simulink model "simcourbe"  (R2018a)
settings: Solver=VariableStepAuto  StartTime=0.0  StopTime=10.0  RelTol=1e-3
undefined symbols (not defined in the file): sigbuilder_block
settings Model: Creator=Raval  LastModifiedBy=Raval

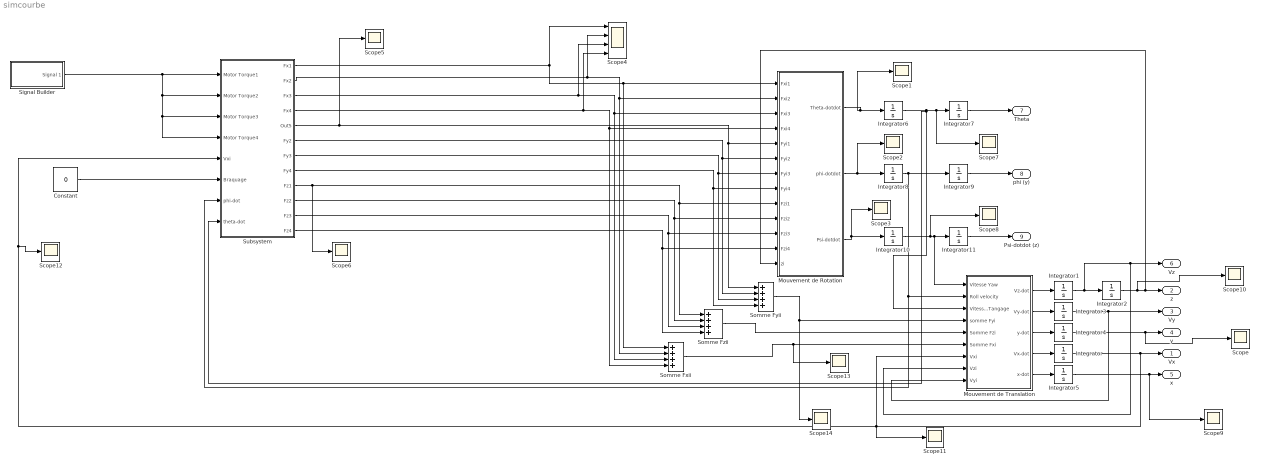
== system simcourbe ==
  Constant : Constant  Value=0  VectorParams1D=off  SampleTime=-1
  Integrator{,1..11} (12 alike) : Integrator
  Mouvement de Rotation : Subsystem
  Mouvement de Translation : Subsystem
  Scope{,1..3,5..14} (14 alike) : Scope
  Scope4 : Scope  NumInputPorts=4
  Signal Builder : Subsystem  Tag=STV Subsys  LoadFcn=sigbuilder_block('load');  StartFcn=sigbuilder_block('start');  StopFcn=sigbuilder_block('stop');  ClipboardFcn=sigbuilder_block('clipboard');  mask(Sigbuilder block){tuvar=[0:10]}
      mask help: Simulink:masks:SigbuilderBlock_MD
      mask init:
      | if ~strcmp(get_param(bdroot(gcbh),'SimulationStatus'),'stopped') tuvar = sigbuilder_block('maskInit'); end
      settings: CopyFcn=sigbuilder_block('copy');  DeleteFcn=sigbuilder_block('delete');  ModelCloseFcn=sigbuilder_block('modelClose');  PreSaveFcn=sigbuilder_block('preSave');  PauseFcn=sigbuilder_block('pause');  ContinueFcn=sigbuilder_block('continue');  NameChangeFcn=sigbuilder_block('namechange');  OpenFcn=sigbuilder_block('open',[366.6 79.8 550.8 400.2 ]);  CloseFcn=sigbuilder_block('close');
      mask Display: plot(0, 0, 100, 100,[2, 2, 32, 32, 2], [68, 8, 8, 68, 68],[32, 2], [38, 38], [32, 19, 2],[53, 60, 44], [32, 17, 17, 2],[16, 16, 31, 31]);txt = getActiveGroup(gcbh);text(2, 100, txt,'verticalAlignment', 'top');
  Somme Fxii : Sum  Inputs=++++
  Somme Fyii : Sum  Inputs=++++
  Somme Fzii : Sum  Inputs=++++
  Subsystem : Subsystem
  Vx : Outport
  z : Outport  Port=2
  Vy : Outport  Port=3
  y : Outport  Port=4
  x : Outport  Port=5
  Vz : Outport  Port=6
  Theta : Outport  Port=7
  phi (y) : Outport  Port=8
  Psi-dotdot (z) : Outport  Port=9
  wires:
  Integrator9/1 -> phi (y)/1
  Subsystem/4(Fx4) -> Scope4/4, Somme Fxii/4, Mouvement de Rotation/4(Fxi4)
  Signal Builder/1(Signal 1) -> Subsystem/1(Motor Torque1), Subsystem/2(Motor Torque2), Subsystem/3(Motor Torque3), Subsystem/4(Motor Torque4)
  Integrator4/1 -> Scope/1, y/1
  Integrator5/1 -> Scope9/1, x/1
  Subsystem/11(Fz3) -> Somme Fzii/3, Mouvement de Rotation/11(Fzi3)
  Subsystem/1(Fx1) -> Mouvement de Rotation/1(Fxi1), Somme Fxii/1, Scope4/1
  Integrator1/1 -> Mouvement de Translation/8(Vzi), Vz/1, Integrator2/1
  Subsystem/3(Fx3) -> Scope4/3, Mouvement de Rotation/3(Fxi3), Somme Fxii/3
  Mouvement de Translation/2(Vy-dot) -> Integrator3/1
  Integrator2/1 -> Scope10/1, Mouvement de Rotation/13(zi), z/1
  Subsystem/5(Out5) -> Scope5/1, Somme Fyii/1, Mouvement de Rotation/5(Fyi1)
  Mouvement de Translation/1(Vz-dot) -> Integrator1/1
  Subsystem/2(Fx2) -> Scope4/2, Somme Fxii/2, Mouvement de Rotation/2(Fxi2)
  Mouvement de Rotation/3(Psi-dotdot) -> Scope3/1, Integrator10/1
  Mouvement de Rotation/1(Theta-dotdot) -> Scope1/1, Integrator6/1
  Subsystem/9(Fz1) -> Scope6/1, Mouvement de Rotation/9(Fzi1), Somme Fzii/1
  Subsystem/6(Fy2) -> Somme Fyii/2, Mouvement de Rotation/6(Fyi2)
  Mouvement de Translation/5(x-dot) -> Integrator5/1
  Somme Fzii/1 -> Mouvement de Translation/5(Somme Fzi)
  Subsystem/10(Fz2) -> Somme Fzii/2, Mouvement de Rotation/10(Fzi2)
  Subsystem/7(Fy3) -> Mouvement de Rotation/7(Fyi3), Somme Fyii/3
  Mouvement de Translation/4(Vx-dot) -> Integrator/1
  Integrator10/1 -> Scope8/1, Mouvement de Translation/1(Vitesse Yaw), Integrator11/1
  Integrator11/1 -> Psi-dotdot (z)/1
  Subsystem/12(Fz4) -> Somme Fzii/4, Mouvement de Rotation/12(Fzi4)
  Integrator8/1 -> Subsystem/7(phi-dot), Mouvement de Translation/2(Roll velocity), Integrator9/1
  Integrator3/1 -> Vy/1, Mouvement de Translation/9(Vyi)
  Mouvement de Translation/3(y-dot) -> Integrator4/1
  Subsystem/8(Fy4) -> Somme Fyii/4, Mouvement de Rotation/8(Fyi4)
  Somme Fyii/1 -> Scope14/1, Mouvement de Translation/4(somme Fyi)
  Integrator7/1 -> Theta/1
  Integrator/1 -> Scope12/1, Subsystem/5(Vxi), Scope11/1, Mouvement de Translation/7(Vxi), Vx/1
  Integrator6/1 -> Subsystem/8(theta-dot), Mouvement de Translation/3(Vitesse Tangage), Scope7/1, Integrator7/1
  Constant/1 -> Subsystem/6(Braquage)
  Mouvement de Rotation/2(phi-dotdot) -> Scope2/1, Integrator8/1
  Somme Fxii/1 -> Scope13/1, Mouvement de Translation/6(Somme Fxi)

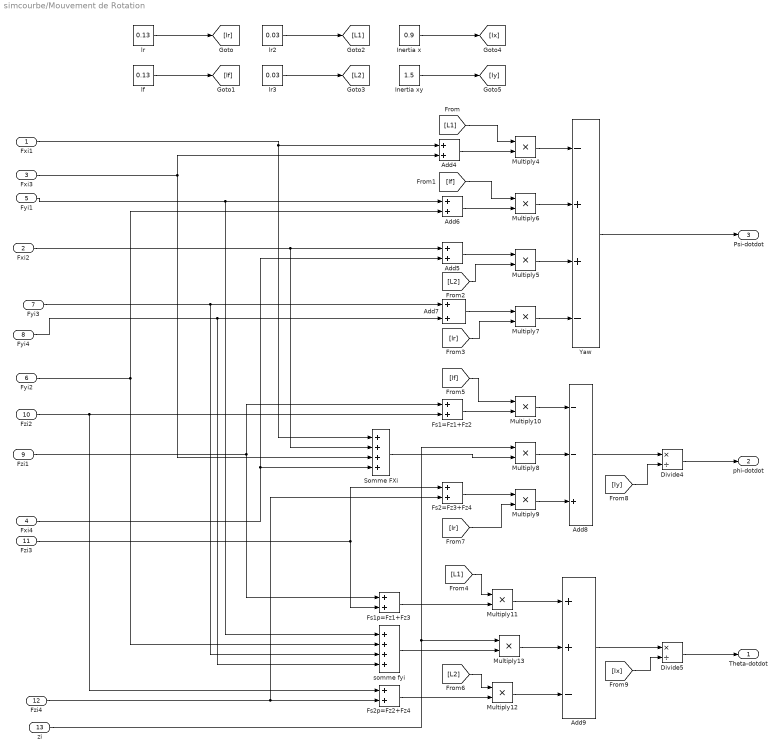
== system simcourbe/Mouvement de Rotation ==
  Fxi1 : Inport
  Fxi2 : Inport  Port=2
  Fxi3 : Inport  Port=3
  Fxi4 : Inport  Port=4
  Fyi1 : Inport  Port=5
  Fyi2 : Inport  Port=6
  Fyi3 : Inport  Port=7
  Fyi4 : Inport  Port=8
  Fzi1 : Inport  Port=9
  Fzi2 : Inport  Port=10
  Fzi3 : Inport  Port=11
  Fzi4 : Inport  Port=12
  zi : Inport  Port=13
  Add{4..7} (4 alike) : Sum
  Add8 : Sum  Inputs=--+
  Add9 : Sum  Inputs=++-
  Divide4 : Product  Inputs=*/
  Divide5 : Product  Inputs=*/
  Fs1=Fz1+Fz2 : Sum
  Fs1p=Fz1+Fz3 : Sum
  Fs2=Fz3+Fz4 : Sum
  Fs2p=Fz2+Fz4 : Sum
  Inertia x : Constant  Value=0.9
  Inertia xy : Constant  Value=1.5
  Multiply{4..13} (10 alike) : Product
  Somme FXi : Sum  Inputs=++++
  Yaw : Sum  Inputs=-++-
  lf : Constant  Value=0.13
  lr : Constant  Value=0.13
  lr2 : Constant  Value=0.03
  lr3 : Constant  Value=0.03
  somme fyi : Sum  Inputs=++++
  Theta-dotdot : Outport
  phi-dotdot : Outport  Port=2
  Psi-dotdot : Outport  Port=3
  wires:
  Add9/1 -> Divide5/1
  Fxi3/1 -> Add4/2, Somme FXi/3
  Yaw/1 -> Psi-dotdot/1
  Multiply9/1 -> Add8/3
  Fxi1/1 -> Somme FXi/1, Add4/1
  zi/1 -> Multiply8/1, Multiply13/1
  Fs2=Fz3+Fz4/1 -> Multiply9/1
  Fyi1/1 -> somme fyi/1, Add6/1
  Fs1p=Fz1+Fz3/1 -> Multiply11/2
  Divide4/1 -> phi-dotdot/1
  Multiply10/1 -> Add8/1
  Add8/1 -> Divide4/1
  Fyi2/1 -> Add6/2, somme fyi/2
  Fxi4/1 -> Add5/2, Somme FXi/4
  Fzi1/1 -> Fs1p=Fz1+Fz3/1, Fs1=Fz1+Fz2/1
  [lr] -> Multiply7/2
  Multiply8/1 -> Add8/2
  Fzi3/1 -> Fs1p=Fz1+Fz3/2, Fs2=Fz3+Fz4/1
  [L2] -> Multiply5/2
  Multiply12/1 -> Add9/3
  Fyi3/1 -> somme fyi/3, Add7/1
  Fxi2/1 -> Somme FXi/2, Add5/1
  [Ix] -> Divide5/2
  somme fyi/1 -> Multiply13/2
  Add5/1 -> Multiply5/1
  Fzi2/1 -> Fs2p=Fz2+Fz4/1, Fs1=Fz1+Fz2/2
  Divide5/1 -> Theta-dotdot/1
  Fyi4/1 -> somme fyi/4, Add7/2
  [lr] -> Multiply9/2
  Fzi4/1 -> Fs2=Fz3+Fz4/2, Fs2p=Fz2+Fz4/2
  [Iy] -> Divide4/2
  Fs1=Fz1+Fz2/1 -> Multiply10/2
  [lf] -> Multiply10/1
  Multiply13/1 -> Add9/2
  Multiply6/1 -> Yaw/2
  Somme FXi/1 -> Multiply8/2
  [L1] -> Multiply11/1
  Fs2p=Fz2+Fz4/1 -> Multiply12/2
  Multiply4/1 -> Yaw/1
  Multiply7/1 -> Yaw/4
  [L2] -> Multiply12/1
  Multiply11/1 -> Add9/1
  Add7/1 -> Multiply7/1
  Multiply5/1 -> Yaw/3
  lr/1 -> [lr]
  lf/1 -> [lf]
  lr2/1 -> [L1]
  lr3/1 -> [L2]
  Inertia x/1 -> [Ix]
  Inertia xy/1 -> [Iy]
  Add4/1 -> Multiply4/2
  [L1] -> Multiply4/1
  Add6/1 -> Multiply6/2
  [lf] -> Multiply6/1

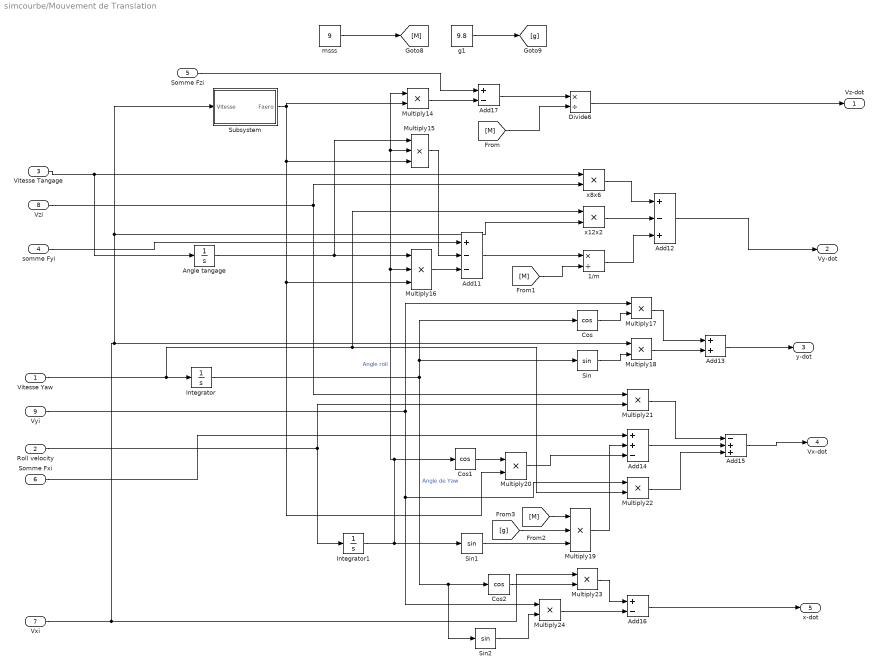
== system simcourbe/Mouvement de Translation ==
  Vitesse Yaw : Inport
  Roll velocity : Inport  Port=2
  Vitesse Tangage : Inport  Port=3
  somme Fyi : Inport  Port=4
  Somme Fzi : Inport  Port=5
  Somme Fxi : Inport  Port=6
  Vxi : Inport  Port=7
  Vzi : Inport  Port=8
  Vyi : Inport  Port=9
  1/m : Product  Inputs=*/
  Add11 : Sum  Inputs=+--
  Add12 : Sum  Inputs=+-+
  Add13 : Sum
  Add14 : Sum  Inputs=++-
  Add15 : Sum  Inputs=-++
  Add16 : Sum  Inputs=+-
  Add17 : Sum  Inputs=+-
  Angle tangage : Integrator
  Cos : Trigonometry  Operator=cos
  Cos1 : Trigonometry  Operator=cos
  Cos2 : Trigonometry  Operator=cos
  Divide6 : Product  Inputs=*/
  Integrator : Integrator
  Integrator1 : Integrator
  Multiply{14,17..18,20..24} (8 alike) : Product
  Multiply15 : Product  Inputs=3
  Multiply16 : Product  Inputs=3
  Multiply19 : Product  Inputs=3
  Sin : Trigonometry
  Sin1 : Trigonometry
  Sin2 : Trigonometry
  Subsystem : Subsystem
  g1 : Constant  Value=9.8
  msss : Constant  Value=9
  x12x2 : Product
  x8x6 : Product
  Vz-dot : Outport
  Vy-dot : Outport  Port=2
  y-dot : Outport  Port=3
  Vx-dot : Outport  Port=4
  x-dot : Outport  Port=5
  wires:
  Vzi/1 -> x8x6/2, Multiply21/1
  Vitesse Yaw/1 -> x12x2/1, Multiply22/2, Integrator/1
  Multiply23/1 -> Add16/1
  Add12/1 -> Vy-dot/1
  Roll velocity/1 -> Multiply21/2, Integrator1/1
  Vyi/1 -> Multiply24/1, Multiply22/1, Multiply17/1
  Add17/1 -> Divide6/1
  somme Fyi/1 -> Add11/1
  Multiply14/1 -> Add17/2
  Subsystem/1(Faero) -> Multiply14/2, Multiply20/2, Multiply16/3, Multiply15/3
  Add15/1 -> Vx-dot/1
  Somme Fzi/1 -> Add17/1
  Integrator/1 -> Sin2/1, Cos2/1, Cos/1, Sin/1  "Angle de Yaw"
  Multiply18/1 -> Add13/2
  Vxi/1 -> Multiply23/1, Subsystem/1(Vitesse), x12x2/2, Multiply18/1
  Integrator1/1 -> Multiply14/1, Multiply15/2, Multiply16/2, Cos1/1, Sin1/1  "Angle roll"
  Add11/1 -> 1/m/1
  Multiply19/1 -> Add14/2
  Multiply24/1 -> Add16/2
  Add14/1 -> Add15/2
  Vitesse Tangage/1 -> Angle tangage/1, x8x6/1
  Angle tangage/1 -> Multiply15/1, Multiply16/1
  Sin2/1 -> Multiply24/2
  Multiply22/1 -> Add15/3
  Add16/1 -> x-dot/1
  Somme Fxi/1 -> Add14/1
  [M] -> Divide6/2
  Multiply16/1 -> Add11/3
  Add13/1 -> y-dot/1
  1/m/1 -> Add12/3
  Divide6/1 -> Vz-dot/1
  Sin/1 -> Multiply18/2
  x12x2/1 -> Add12/2
  Cos/1 -> Multiply17/2
  Multiply17/1 -> Add13/1
  Cos1/1 -> Multiply20/1
  Multiply20/1 -> Add14/3
  Multiply15/1 -> Add11/2
  x8x6/1 -> Add12/1
  Cos2/1 -> Multiply23/2
  Multiply21/1 -> Add15/1
  Sin1/1 -> Multiply19/3
  [g] -> Multiply19/2
  msss/1 -> [M]
  [M] -> 1/m/2
  [M] -> Multiply19/1
  g1/1 -> [g]

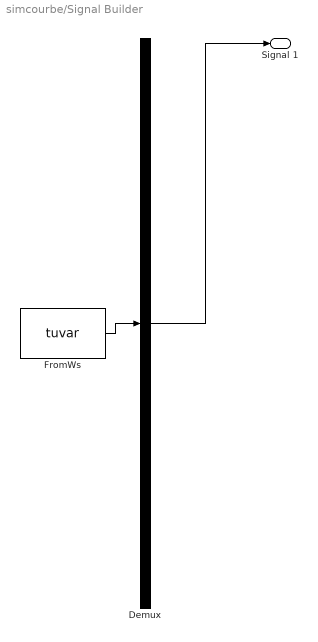
== system simcourbe/Signal Builder ==
  Demux : Demux  Tag=STV Demux  Outputs=1
  FromWs : FromWorkspace  Tag=STV FromWs  VariableName=tuvar  SampleTime=0
      SigBuilderData=|
      | common.afterFinalStr = 'Extrapolate'
      | common.sampleTime = 0
      | dataSet.timeRange = [0 10]
      | dataSet.name = 'Group 1'
      | sbobj.Groups.Name = 'Group 1'
      | sbobj.Groups.Signals.Name = 'Signal 1'
      | sbobj.Groups.Signals.XData = [0 4 4 6 6 10]
      | sbobj.Groups.Signals.YData = [0 0.995 1 1 0.995 0.995]
  Signal 1 : Outport  Tag=STV Outport
  wires:
  Demux/1 -> Signal 1/1
  FromWs/1 -> Demux/1

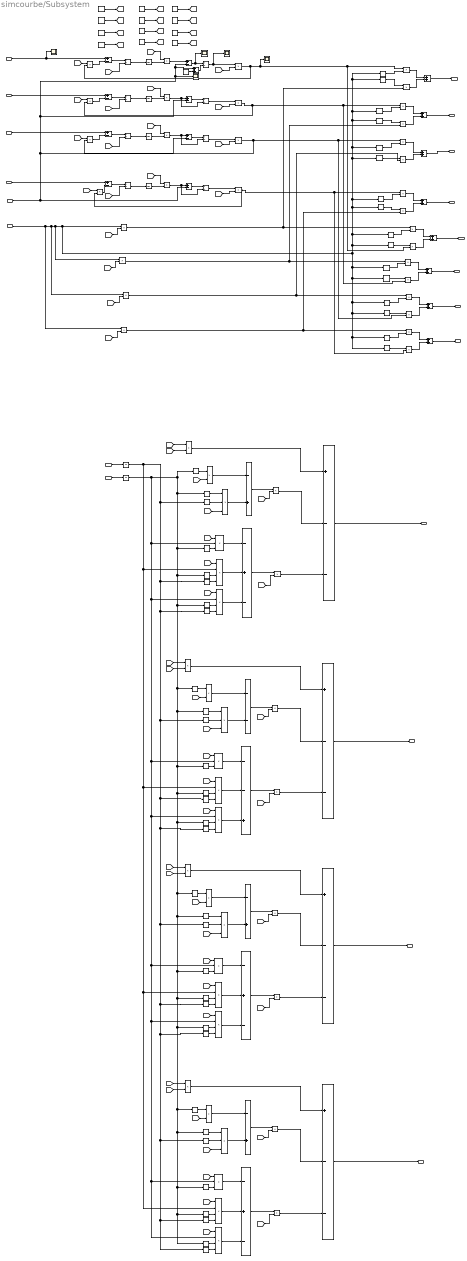
== system simcourbe/Subsystem ==
  Motor Torque1 : Inport
  Motor Torque2 : Inport  Port=2
  Motor Torque3 : Inport  Port=3
  Motor Torque4 : Inport  Port=4
  Vxi : Inport  Port=5
  Braquage : Inport  Port=6
  phi-dot : Inport  Port=7
  theta-dot : Inport  Port=8
  Add{,5..11,24} (9 alike) : Sum
  Add{1..4} (4 alike) : Sum  Inputs=+-
  Add12 : Sum  Inputs=-+
  Add13 : Sum  Inputs=-+-
  Add{14,17,20,23} (4 alike) : Sum  Inputs=+--
  Add15 : Sum  Inputs=--
  Add16 : Sum  Inputs=--+
  Add18 : Sum  Inputs=-+
  Add19 : Sum  Inputs=-+-
  Add21 : Sum  Inputs=-+
  Add22 : Sum  Inputs=-+-
  Coefficient Fx : Constant  Value=0.1
  Constant : Constant  Value=0.1
  Constant1 : Constant  Value=0.5
  Constant2 : Constant  Value=0.000001
  Cos{,1..11,14..15,18..21,24..27,30..31} (24 alike) : Trigonometry  Operator=cos
  Cos{12..13,16..17,22..23,28..29} (8 alike) : Trigonometry
  Divide{2..9} (8 alike) : Product  Inputs=*/
  Inertia Roue : Constant  Value=0.2
  Integrator : Integrator
  Integrator12 : Integrator
  Integrator14 : Integrator  InitialCondition=0.001
  Integrator15 : Integrator  InitialCondition=0.001
  Integrator16 : Integrator  InitialCondition=0.001
  Integrator17 : Integrator
  Kvi : Constant
  L1 : Constant  Value=0.03
  L2 : Constant  Value=0.03
  Multiply{,1..24,26,30..32,34,38..40,42,46..48,50,54..59} (44 alike) : Product
  Multiply{25,27,33,35,41,43,49,51} (8 alike) : Product  Inputs=3
  Multiply{28..29,36..37,44..45,52..53} (8 alike) : Product  Inputs=4
  Rayon : Constant  Value=0.031
  Rw-vx{1..4} (4 alike) : Sum  Inputs=+-
  Rw{1..4} (4 alike) : Product
  Scope{,1..2,4..5} (5 alike) : Scope
  Sin{,1..15} (16 alike) : Trigonometry
  g : Constant  Value=9.8
  ksi : Constant
  lf : Constant  Value=0.13
  lr : Constant  Value=0.13
  Fx1 : Outport
  Fx2 : Outport  Port=2
  Fx3 : Outport  Port=3
  Fx4 : Outport  Port=4
  Out5 : Outport  Port=5
  Fy2 : Outport  Port=6
  Fy3 : Outport  Port=7
  Fy4 : Outport  Port=8
  Fz1 : Outport  Port=9
  Fz2 : Outport  Port=10
  Fz3 : Outport  Port=11
  Fz4 : Outport  Port=12
  wires:
  Integrator17/1 -> Multiply53/2, Multiply51/2, Multiply45/2, Multiply43/2, Multiply37/2, Multiply35/2, Multiply29/2, Multiply27/2, Cos9/1, Cos28/1, Cos26/1, Cos31/1, Cos30/1, Sin14/1, Cos22/1, Cos20/1, Cos25/1, Cos24/1, Sin12/1, Cos16/1, Cos14/1, Cos19/1, Cos18/1, Sin10/1, Cos12/1, Cos10/1, Cos8/1, Sin8/1
  Multiply12/1 -> Add6/1
  Integrator12/1 -> Multiply52/2, Multiply44/2, Multiply36/2, Multiply28/2, Cos11/1, Cos13/1, Cos15/1, Cos17/1, Cos21/1, Cos23/1, Cos29/1, Cos27/1, Sin15/1, Sin13/1, Sin11/1, Sin9/1
  Add8/1 -> Out5/1
  Sin9/1 -> Multiply25/2
  Add4/1 -> Divide8/1
  Multiply35/1 -> Add16/1
  Divide4/1 -> Integrator14/1
  [Cy] -> Multiply6/2
  Vxi/1 -> Rw-vx4/2, Rw-vx2/2, Add24/1, Rw-vx1/2, Scope2/1, Rw-vx3/2
  Rw-vx2/1 -> Divide5/1
  Braquage/1 -> Multiply7/1, Multiply6/1, Multiply5/1, Sin3/1, Cos/1, Sin/1, Cos1/1, Sin1/1, Cos2/1, Sin2/1, Cos3/1, Cos4/1, Sin4/1, Sin7/1, Cos7/1, Sin6/1, Cos6/1, Sin5/1, Cos5/1, Multiply/1
  Multiply8/1 -> Add/1
  Multiply55/1 -> Add23/2
  Add6/1 -> Fx3/1
  Cos24/1 -> Multiply41/1
  [Cx] -> Multiply3/2
  Add13/1 -> Multiply30/1
  [L2] -> Multiply37/1
  Cos17/1 -> Multiply37/4
  Constant1/1 -> [M]
  Sin/1 -> Multiply9/1
  Sin14/1 -> Multiply50/1
  Rw2/1 -> Divide5/2, Rw-vx2/1
  Multiply18/1 -> Add9/1
  Multiply22/1 -> Add11/1
  Divide8/1 -> Integrator16/1
  Sin7/1 -> Multiply23/1
  Integrator15/1 -> Rw3/2
  Cos30/1 -> Multiply49/1
  Add/1 -> Fx1/1
  Sin1/1 -> Multiply11/1
  Cos2/1 -> Multiply12/2
  Integrator16/1 -> Rw4/2
  Cos6/1 -> Multiply20/2
  L2/1 -> [L2]
  [L1] -> Multiply45/1
  Multiply45/1 -> Add19/3
  Integrator14/1 -> Rw2/2
  Cos3/1 -> Multiply14/2
  [R] -> Rw3/1
  Multiply10/1 -> Add5/1
  Divide9/1 -> Multiply4/1
  Sin10/1 -> Multiply34/1
  Add20/1 -> Fz3/1
  Multiply51/1 -> Add22/1
  [L1] -> Multiply28/1
  Multiply1/1 -> Multiply56/2, Scope1/1, Multiply17/2, Multiply8/1  "Fxpi"
  [Cy] -> Multiply/2
  Add17/1 -> Fz2/1
  Add23/1 -> Fz4/1
  Multiply27/1 -> Add13/1
  Rw4/1 -> Divide9/2, Rw-vx4/1
  [M] -> Multiply48/2
  Multiply7/1 -> Multiply22/1, Multiply15/2  "Fypi"
  Motor Torque2/1 -> Add2/1
  Multiply24/1 -> Add14/1
  theta-dot/1 -> Integrator12/1
  Kvi/1 -> [kvi]
  phi-dot/1 -> Integrator17/1
  Rayon/1 -> [R]
  [Ir] -> Divide8/2
  [Cy] -> Multiply7/2
  Constant/1 -> [Cy]
  Integrator/1 -> Rw1/2
  Cos11/1 -> Multiply28/4
  Add5/1 -> Fx2/1
  Add14/1 -> Fz1/1
  Cos7/1 -> Multiply22/2
  Rw3/1 -> Divide7/2, Rw-vx3/1
  Divide7/1 -> Multiply3/1
  [R] -> Rw1/1
  ksi/1 -> [ksi]
  Rw-vx1/1 -> Scope5/1, Divide3/1
  Sin5/1 -> Multiply19/1
  [Ir] -> Divide2/2
  [ksi] -> Multiply55/2
  Divide3/1 -> Scope4/1, Multiply1/1
  [R] -> Rw2/1
  Multiply/1 -> Multiply16/1, Multiply9/2  "Fypi"
  Inertia Roue/1 -> [Ir]
  Multiply17/1 -> Add8/2
  Cos18/1 -> Multiply33/1
  Rw-vx3/1 -> Divide7/1
  Multiply13/1 -> Add6/2
  Multiply54/1 -> Add23/3
  [kvi] -> Multiply46/2
  Multiply44/1 -> Add19/2
  Motor Torque3/1 -> Add3/1
  Rw-vx4/1 -> Divide9/1
  Multiply30/1 -> Add14/3
  Add22/1 -> Multiply54/1
  Cos13/1 -> Multiply29/4
  Add7/1 -> Fx4/1
  [ksi] -> Multiply31/2
  Multiply21/1 -> Add10/2
  Multiply47/1 -> Add20/2
  Add1/1 -> Divide2/1
  [lf] -> Multiply27/1
  Cos28/1 -> Multiply53/3
  Cos29/1 -> Multiply53/4
  Multiply6/1 -> Multiply20/1, Multiply13/2  "Fypi"
  Multiply11/1 -> Add5/2
  Cos20/1 -> Multiply44/3
  [Cx] -> Multiply2/2
  [L2] -> Multiply52/1
  L1/1 -> [L1]
  Cos23/1 -> Multiply45/4
  Cos26/1 -> Multiply52/3
  Multiply28/1 -> Add13/2
  Multiply16/1 -> Add8/1
  Cos9/1 -> Multiply27/3
  Cos5/1 -> Multiply18/2
  Add15/1 -> Multiply39/1
  Cos10/1 -> Multiply28/3
  Cos19/1 -> Multiply35/3
  Cos16/1 -> Multiply37/3
  [lf] -> Multiply35/1
  lf/1 -> [lf]
  Multiply31/1 -> Add14/2
  [kvi] -> Multiply38/2
  [L1] -> Multiply25/3
  Sin3/1 -> Multiply15/1
  Multiply32/1 -> Add17/1
  [Cx] -> Multiply4/2
  Multiply38/1 -> Add17/3
  Cos31/1 -> Multiply51/3
  Multiply37/1 -> Add16/3
  Coefficient Fx/1 -> [Cx]
  Sin4/1 -> Multiply17/1
  Multiply19/1 -> Add9/2
  Sin11/1 -> Multiply33/2
  [L2] -> Multiply49/3
  Add10/1 -> Fy3/1
  [R] -> Rw4/1
  Multiply5/1 -> Multiply18/1, Multiply11/2  "Fypi"
  [ksi] -> Multiply39/2
  Multiply29/1 -> Add13/3
  Multiply23/1 -> Add11/2
  [M] -> Multiply32/2
  [kvi] -> Multiply30/2
  Multiply36/1 -> Add16/2
  Multiply39/1 -> Add17/2
  [M] -> Multiply40/2
  [Ir] -> Divide6/2
  Motor Torque4/1 -> Add4/1
  [g] -> Multiply40/1
  [L1] -> Multiply41/3
  [lr] -> Multiply42/2
  Sin6/1 -> Multiply21/1
  Cos15/1 -> Multiply36/4
  Divide2/1 -> Integrator/1
  Add12/1 -> Multiply31/1
  [L1] -> Multiply29/1
  Multiply34/1 -> Add15/1
  Multiply48/1 -> Add23/1
  Sin12/1 -> Multiply42/1
  Multiply46/1 -> Add20/3
  [Ir] -> Divide4/2
  Sin13/1 -> Multiply41/2
  Multiply41/1 -> Add18/2
  [Cy] -> Multiply5/2
  Multiply42/1 -> Add18/1
  Cos25/1 -> Multiply43/3
  Add2/1 -> Divide4/1
  Cos4/1 -> Multiply16/2
  [L2] -> Multiply33/3
  [lf] -> Multiply43/1
  Multiply40/1 -> Add20/1
  Cos21/1 -> Multiply44/4
  Cos12/1 -> Multiply29/3
  [ksi] -> Multiply47/2
  [L2] -> Multiply53/1
  Cos14/1 -> Multiply36/3
  [g] -> Multiply48/1
  Multiply20/1 -> Add10/1
  Divide5/1 -> Multiply2/1
  Cos22/1 -> Multiply45/3
  Add3/1 -> Divide6/1
  [L2] -> Multiply36/1
  [L1] -> Multiply44/1
  Multiply53/1 -> Add22/3
  Add18/1 -> Multiply47/1
  Multiply50/1 -> Add21/1
  Multiply49/1 -> Add21/2
  [lr] -> Multiply50/2
  [kvi] -> Multiply54/2
  Sin15/1 -> Multiply49/2
  lr/1 -> [lr]
  [g] -> Multiply32/1
  Add21/1 -> Multiply55/1
  Multiply33/1 -> Add15/2
  Multiply15/1 -> Add7/2
  Add16/1 -> Multiply38/1
  Add19/1 -> Multiply46/1
  [lf] -> Multiply51/1
  Multiply43/1 -> Add19/1
  [lf] -> Multiply34/2
  [Cx] -> Multiply1/2
  Divide6/1 -> Integrator15/1
  Cos8/1 -> Multiply25/1
  Multiply52/1 -> Add22/2
  Multiply9/1 -> Add/2
  Cos27/1 -> Multiply52/4
  Multiply25/1 -> Add12/2
  Multiply14/1 -> Add7/1
  Cos1/1 -> Multiply10/2
  Cos/1 -> Multiply8/2
  Add11/1 -> Fy4/1
  Sin2/1 -> Multiply13/1
  Add9/1 -> Fy2/1
  [M] -> Multiply24/2
  Multiply26/1 -> Add12/1
  [g] -> Multiply24/1
  g/1 -> [g]
  Sin8/1 -> Multiply26/1
  [lf] -> Multiply26/2
  Motor Torque1/1 -> Scope/1, Add1/1
  Multiply56/1 -> Add1/2
  [R] -> Multiply56/1
  [R] -> Multiply57/1
  Multiply57/1 -> Add2/2
  Multiply2/1 -> Multiply57/2, Multiply19/2, Multiply10/1  "Fxpi"
  [R] -> Multiply58/1
  Multiply58/1 -> Add3/2
  Multiply3/1 -> Multiply58/2, Multiply21/2, Multiply12/1  "Fxpi"
  [R] -> Multiply59/1
  Multiply59/1 -> Add4/2
  Multiply4/1 -> Multiply59/2, Multiply23/2, Multiply14/1  "Fxpi"
  Rw1/1 -> Rw-vx1/1
  Constant2/1 -> Add24/2
  Add24/1 -> Divide3/2

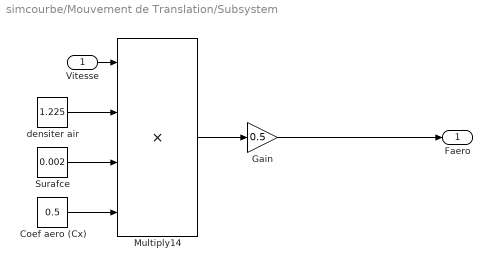
== system simcourbe/Mouvement de Translation/Subsystem ==
  Vitesse : Inport
  Coef aero (Cx) : Constant  Value=0.5
  Gain : Gain  Gain=0.5
  Multiply14 : Product  Inputs=4
  Surafce : Constant  Value=0.002
  densiter air : Constant  Value=1.225
  Faero : Outport
  wires:
  Vitesse/1 -> Multiply14/1
  densiter air/1 -> Multiply14/2
  Surafce/1 -> Multiply14/3
  Coef aero (Cx)/1 -> Multiply14/4
  Multiply14/1 -> Gain/1
  Gain/1 -> Faero/1
